simulink model "pitchHresponse"  (R2021a)
settings: Solver=VariableStepAuto  StartTime=0.0  StopTime=30  RelTol=1e-3
settings Model: Creator=pedro  LastModifiedBy=pedro
settings DataIOCC: ReturnWorkspaceOutputs=off

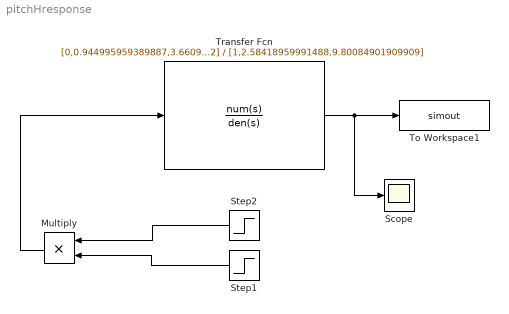
== system pitchHresponse ==
  Multiply : Product
  Scope : Scope
  Step1 : Step  Time=15  After=0.2  SampleTime=1
  Step2 : Step  Time=18  Before=1  After=0  SampleTime=1
  To Workspace1 : ToWorkspace  VariableName=simout  SaveFormat=Structure With Time  SampleTime=0.065
  Transfer Fcn : TransferFcn  Numerator=[0,0.944995959389887,3.66094198989342]  Denominator=[1,2.58418959991488,9.80084901909909]
  wires:
  Step1/1 -> Multiply/2
  Step2/1 -> Multiply/1
  Multiply/1 -> Transfer Fcn/1
  Transfer Fcn/1 -> To Workspace1/1, Scope/1
